simulink model "hw10ch"  (R2013a)
settings: Solver=ode45  StartTime=0.0  StopTime=10.0  RelTol=1e-3
settings Model: Creator=bazkoale  LastModifiedBy=bazkoale

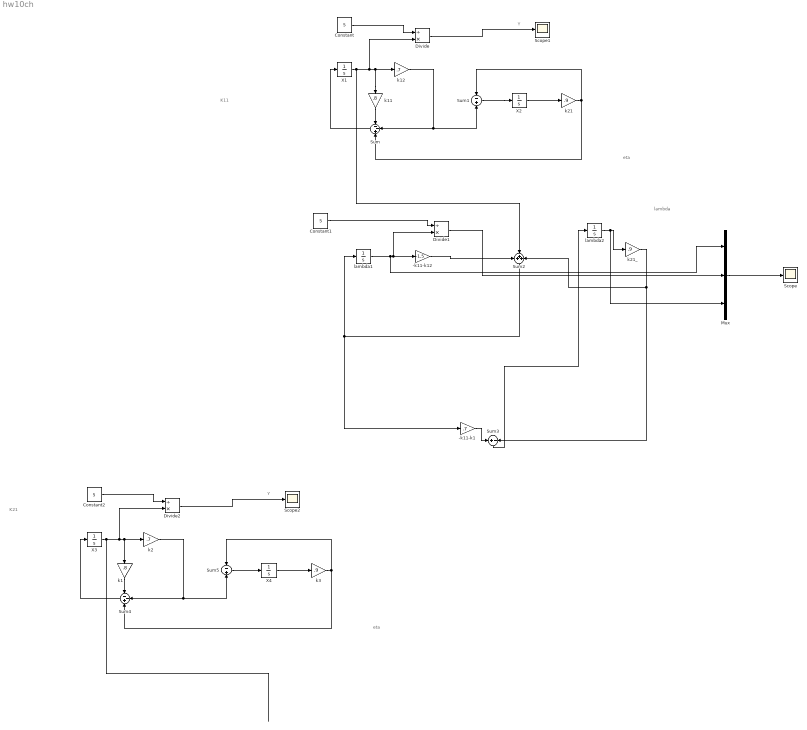
== system hw10ch ==
  note: K21
  note: Y
  note: lambda
  note: eta
  note: K11
  note: Y
  note: eta
  -k11-k1 : Gain  Gain=.7
  -k11-k12 : Gain  Gain=-1.5
  Constant : Constant  Value=5
  Constant1 : Constant  Value=5
  Constant2 : Constant  Value=5
  Divide : Product  Inputs=/*
  Divide1 : Product  Inputs=/*
  Divide2 : Product  Inputs=/*
  Mux : Mux  Inputs=3
  Scope : Scope
  Scope1 : Scope
  Scope2 : Scope
      settings: SaveName=ScopeData2
  Sum : Sum  Inputs=--+
  Sum1 : Sum  Inputs=-+
  Sum2 : Sum  Inputs=+++
  Sum3 : Sum  Inputs=+-
  Sum4 : Sum  Inputs=--+
  Sum5 : Sum  Inputs=-+
  X1 : Integrator  InitialCondition=200
  X2 : Integrator
  X3 : Integrator  InitialCondition=200
  X4 : Integrator
  k1 : Gain  Gain=.8
  k11 : Gain  Gain=.8
  k12 : Gain  Gain=.7
  k2 : Gain  Gain=.7
  k21 : Gain  Gain=.9
  k21_ : Gain  Gain=.9
  k3 : Gain  Gain=.9
  lambda1 : Integrator
  lambda2 : Integrator
  wires:
  X1/1 -> Divide/2, k11/1, k12/1, Sum2/2
  k12/1 -> Sum1/2, Sum/2
  Sum/1 -> X1/1
  X2/1 -> k21/1
  Sum1/1 -> X2/1
  k21/1 -> Sum1/1, Sum/3
  k11/1 -> Sum/1
  Constant/1 -> Divide/1
  lambda1/1 -> Mux/1, Divide1/2, -k11-k12/1
  -k11-k12/1 -> Sum2/1
  lambda2/1 -> Mux/3, k21_/1
  k21_/1 -> Sum3/2, Sum2/3
  Mux/1 -> Scope/1
  Constant1/1 -> Divide1/1
  Divide1/1 -> Mux/2
  Divide/1 -> Scope1/1
  Sum2/1 -> lambda1/1, -k11-k1/1
  -k11-k1/1 -> Sum3/1
  Sum3/1 -> lambda2/1
  X3/1 -> k2/1, k1/1, Divide2/2
  k2/1 -> Sum4/2, Sum5/2
  Sum4/1 -> X3/1
  X4/1 -> k3/1
  Sum5/1 -> X4/1
  k3/1 -> Sum4/3, Sum5/1
  k1/1 -> Sum4/1
  Constant2/1 -> Divide2/1
  Divide2/1 -> Scope2/1
